simulink model "Q7_simulation"  (R2017b)
settings: Solver=VariableStepAuto  StartTime=0.0  StopTime=50  RelTol=1e-3
settings Model: Creator=HeMaTshop  LastModifiedBy=HeMaTshop

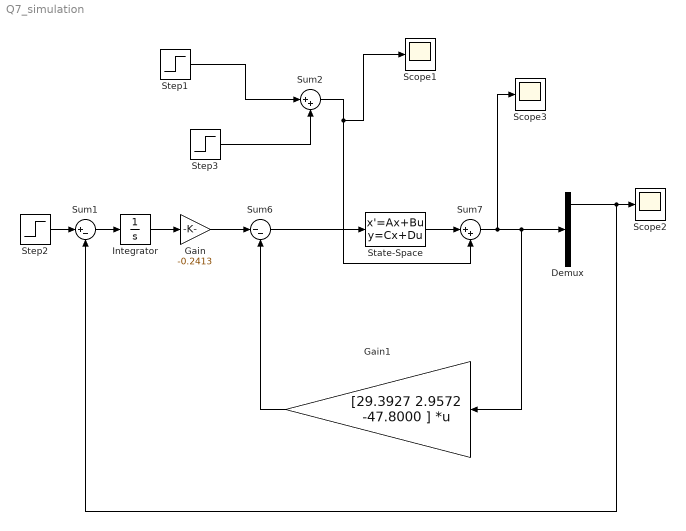
== system Q7_simulation ==
  Demux : Demux  Outputs=3
  Gain : Gain  Gain=-0.2413
  Gain1 : Gain  Gain="[29.3927    2.9572  -47.8000 ]"  Multiplication=Matrix(K*u)
  Integrator : Integrator
  Scope1 : Scope
  Scope2 : Scope
  Scope3 : Scope
  State-Space : StateSpace  A=[0 1 0;9.8/0.03 0 24.8656;0 0 -250]  B=[0;0;5]  C=eye(3)  D=[0;0;0]  InitialCondition=0
  Step1 : Step  Time=20  SampleTime=0
  Step2 : Step  Time=0  SampleTime=0
  Step3 : Step  Time=21  After=-1  SampleTime=0
  Sum1 : Sum  Inputs=|+-
  Sum2 : Sum  Inputs=|++
  Sum6 : Sum  Inputs=|--
  Sum7 : Sum  Inputs=|++
  wires:
  State-Space/1 -> Sum7/1
  Sum6/1 -> State-Space/1
  Sum7/1 -> Scope3/1, Gain1/1, Demux/1
  Gain1/1 -> Sum6/2
  Integrator/1 -> Gain/1
  Gain/1 -> Sum6/1
  Step2/1 -> Sum1/1
  Sum1/1 -> Integrator/1
  Demux/1 -> Sum1/2, Scope2/1
  Step3/1 -> Sum2/2
  Step1/1 -> Sum2/1
  Sum2/1 -> Sum7/2, Scope1/1
